simulink model "Day1_model"  (R2022b)
settings: Solver=ode4  StartTime=0.0  StopTime=10.0  FixedStep=0.001  RelTol=1e-3
values from neighbouring files (symbols this model uses):
  A_ss = [0 1; -K/M -D/M]    [Day1.m]
  B_ss = [0; 1/M]    [Day1.m]
  C_ss = [1 0]    [Day1.m]
  D = 3    [Day1.m]    (also in Day1_3.m = 1)
  D_ss = [0]    [Day1.m]
  K = 10    [Day1.m]    (also in Day1_3.m)
  M = 1    [Day1.m]    (also in Day1_3.m = 10)
settings Model: Creator=user  LastModifiedBy=user

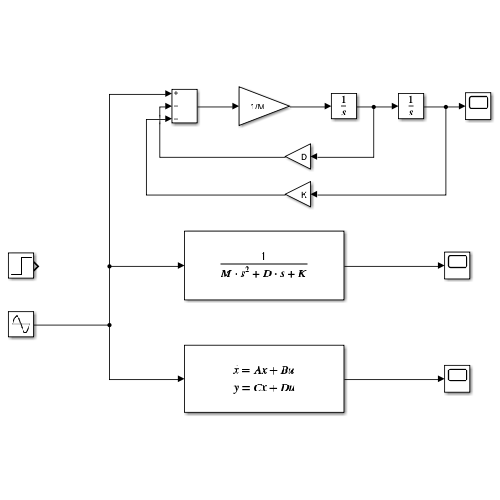
[thumbnail: Simulink's stored preview of the top-level diagram]
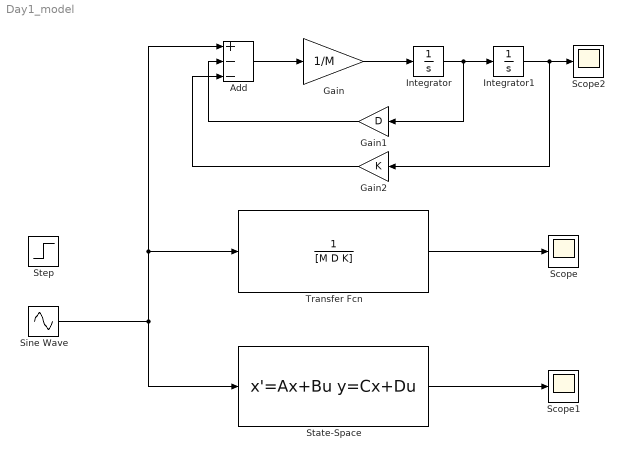
== system Day1_model ==
  Add : Sum  Inputs=+--
  Gain : Gain  Gain=1/M
  Gain1 : Gain  Gain=D
  Gain2 : Gain  Gain=K
  Integrator : Integrator
  Integrator1 : Integrator
  Scope : Scope
  Scope1 : Scope
  Scope2 : Scope
  Sine Wave : Sin  SampleTime=0
  State-Space : StateSpace  A=A_ss  B=B_ss  C=C_ss  D=D_ss  InitialCondition=0
  Step : Step  SampleTime=0
  Transfer Fcn : TransferFcn  Denominator=[M D K]
  wires:
  Transfer Fcn/1 -> Scope/1
  State-Space/1 -> Scope1/1
  Add/1 -> Gain/1
  Gain/1 -> Integrator/1
  Integrator/1 -> Gain1/1, Integrator1/1
  Integrator1/1 -> Gain2/1, Scope2/1
  Gain1/1 -> Add/2
  Gain2/1 -> Add/3
  Sine Wave/1 -> Add/1, Transfer Fcn/1, State-Space/1
